simulink model "B1_quadcopter_model"  (R2021b)
settings: Solver=VariableStepAuto  StartTime=0.0  StopTime=10  RelTol=1e-3
values from neighbouring files (symbols this model uses):
  K_act = 50    [A10_simple_plant.m]    (also in A11_setup_script_pprz.m = 20; A1_setup_script.m = 20)
  K_act_inner = K_act*eye(4)    [A11_setup_script_pprz.m]    (also in A1_setup_script.m)
  K_u_d = 2.5    [A11_setup_script_pprz.m]    (also in A1_setup_script.m = 7)
  K_v_d = 2.5    [A11_setup_script_pprz.m]    (also in A1_setup_script.m = 7)
  K_w_d = 2.5    [A11_setup_script_pprz.m]    (also in A1_setup_script.m = 7)
  max_motor_rate = 30000    [A11_setup_script_pprz.m]    (also in A1_setup_script.m)
  max_omega_motor = 11000    [A11_setup_script_pprz.m]    (also in A1_setup_script.m)
  omega_c_motors = 50    [A11_setup_script_pprz.m]    (also in A1_setup_script.m)
  sampling_time = 1/frequency    (= 0.002)    [A11_setup_script_pprz.m]    (also in A12_sim_multi_run.m; A1_setup_script.m; A6_slow_actuator.m)
undefined symbols (not defined in the file or in its folder): K_ec_d_p, K_ec_d_q, K_ec_d_r, K_ec_dd_p, K_ec_dd_q, K_ec_dd_r, K_ec_p, K_ec_q, K_ec_r, K_p, K_p_d, K_p_dd, K_q, K_q_d, K_q_dd, K_r, K_r_d, K_r_dd
libraries: dspinverses x11, simulink_extras x6, sim3dlib x1, uavsim3dlib x1, vrlib x1, aerolibutil x1, sharedutil x1, aerolibbdyn x1, aerolibatmos2 x1
(part 1 of 3)
settings Model: Creator=pieca  LastModifiedBy=pieca

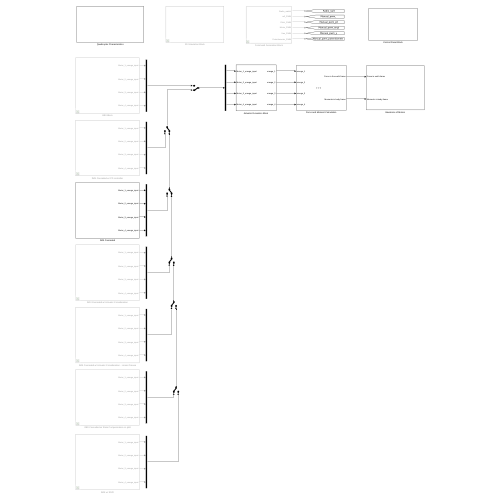
[thumbnail: Simulink's stored preview of the top-level diagram]
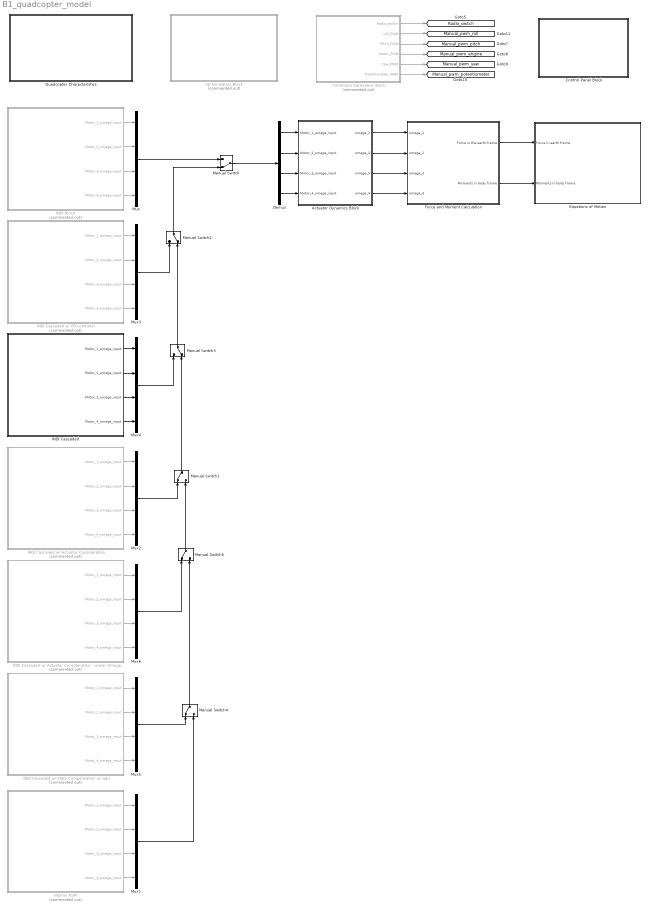
== system B1_quadcopter_model ==
  3D Simulation Block : Subsystem  Commented=on
  Actuator Dynamics Block : Subsystem
  Command Generation Block : Subsystem  Commented=on
  Control Panel Block : Subsystem
  Demux : Demux
  Equations of Motion : Subsystem
  Force and Moment Calculation : Subsystem
      mask Display: image('C:\Users\pieca\Desktop\AE5310-Thesis-Control\Quadcopter\media\bebop.jpg'); % Use "Edit Image" on toolstrip to change.
  INDI Block : Subsystem  Commented=on
  INDI Cascaded : Subsystem
  INDI Cascaded w/ Actuator Consideration : Subsystem  Commented=on
  INDI Cascaded w/ Actuator Consideration - Linear Omega : Subsystem  Commented=on
  INDI Cascaded w/ PD controller : Subsystem  Commented=on
  INDI Cascaded w/ State Compensation on qdd : Subsystem  Commented=on
  INDI w/ RSPI : Subsystem  Commented=on
  Manual Switch : ManualSwitch  CurrentSetting=0
  Manual Switch1 : ManualSwitch
  Manual Switch2 : ManualSwitch  CurrentSetting=0
  Manual Switch3 : ManualSwitch  CurrentSetting=0
  Manual Switch4 : ManualSwitch
  Manual Switch5 : ManualSwitch
  Mux{,1..6} (7 alike) : Mux
  Quadcopter Characteristics : Subsystem
  tag scope: Manual_pwm_engine=global, Manual_pwm_pitch=global, Manual_pwm_potentiometer=global, Manual_pwm_roll=global, Manual_pwm_yaw=global, Radio_switch=global
  wires:
  Command Generation Block/1(Radio_switch) -> [Radio_switch]
  Command Generation Block/2(roll_PWM) -> [Manual_pwm_roll]
  Command Generation Block/3(Pitch_PWM) -> [Manual_pwm_pitch]
  Command Generation Block/4(Motor_PWM) -> [Manual_pwm_engine]
  Command Generation Block/5(Yaw_PWM) -> [Manual_pwm_yaw]
  Command Generation Block/6(Potentiometer_PWM) -> [Manual_pwm_potentiometer]
  INDI Block/1(Motor_1_omega_input) -> Mux/1
  INDI Block/2(Motor_2_omega_input) -> Mux/2
  INDI Block/3(Motor_3_omega_input) -> Mux/3
  INDI Block/4(Motor_4_omega_input) -> Mux/4
  Demux/1 -> Actuator Dynamics Block/1(Motor_1_omega_input)
  Demux/2 -> Actuator Dynamics Block/2(Motor_2_omega_input)
  Demux/3 -> Actuator Dynamics Block/3(Motor_3_omega_input)
  Demux/4 -> Actuator Dynamics Block/4(Motor_4_omega_input)
  Force and Moment Calculation/1(Force in the earth frame) -> Equations of Motion/1(Force in earth frame)
  Force and Moment Calculation/2(Moments in body frame) -> Equations of Motion/2(Moments in body frame)
  Actuator Dynamics Block/1(omega_1) -> Force and Moment Calculation/1(omega_1)
  Actuator Dynamics Block/2(omega_2) -> Force and Moment Calculation/2(omega_2)
  Actuator Dynamics Block/3(omega_3) -> Force and Moment Calculation/3(omega_3)
  Actuator Dynamics Block/4(omega_4) -> Force and Moment Calculation/4(omega_4)
  INDI w/ RSPI/3(Motor_3_omega_input) -> Mux1/3
  INDI w/ RSPI/4(Motor_4_omega_input) -> Mux1/4
  INDI w/ RSPI/2(Motor_2_omega_input) -> Mux1/2
  INDI w/ RSPI/1(Motor_1_omega_input) -> Mux1/1
  Mux/1 -> Manual Switch/1
  Manual Switch/1 -> Demux/1
  INDI Cascaded w/ Actuator Consideration/4(Motor_4_omega_input) -> Mux2/4
  INDI Cascaded w/ Actuator Consideration/1(Motor_1_omega_input) -> Mux2/1
  INDI Cascaded w/ Actuator Consideration/2(Motor_2_omega_input) -> Mux2/2
  INDI Cascaded w/ Actuator Consideration/3(Motor_3_omega_input) -> Mux2/3
  Mux2/1 -> Manual Switch1/1
  INDI Cascaded w/ PD controller/2(Motor_2_omega_input) -> Mux3/2
  INDI Cascaded w/ PD controller/3(Motor_3_omega_input) -> Mux3/3
  INDI Cascaded w/ PD controller/1(Motor_1_omega_input) -> Mux3/1
  INDI Cascaded w/ PD controller/4(Motor_4_omega_input) -> Mux3/4
  Manual Switch2/1 -> Manual Switch/2
  Mux3/1 -> Manual Switch2/1
  INDI Cascaded/4(Motor_4_omega_input) -> Mux4/4
  INDI Cascaded/3(Motor_3_omega_input) -> Mux4/3
  INDI Cascaded/2(Motor_2_omega_input) -> Mux4/2
  INDI Cascaded/1(Motor_1_omega_input) -> Mux4/1
  Manual Switch1/1 -> Manual Switch3/2
  Manual Switch3/1 -> Manual Switch2/2
  Mux4/1 -> Manual Switch3/1
  INDI Cascaded w/ State Compensation on qdd/3(Motor_3_omega_input) -> Mux5/3
  INDI Cascaded w/ State Compensation on qdd/4(Motor_4_omega_input) -> Mux5/4
  INDI Cascaded w/ State Compensation on qdd/1(Motor_1_omega_input) -> Mux5/1
  INDI Cascaded w/ State Compensation on qdd/2(Motor_2_omega_input) -> Mux5/2
  Mux5/1 -> Manual Switch4/1
  Mux1/1 -> Manual Switch4/2
  INDI Cascaded w/ Actuator Consideration - Linear Omega/2(Motor_2_omega_input) -> Mux6/2
  INDI Cascaded w/ Actuator Consideration - Linear Omega/4(Motor_4_omega_input) -> Mux6/4
  INDI Cascaded w/ Actuator Consideration - Linear Omega/3(Motor_3_omega_input) -> Mux6/3
  INDI Cascaded w/ Actuator Consideration - Linear Omega/1(Motor_1_omega_input) -> Mux6/1
  Mux6/1 -> Manual Switch5/1
  Manual Switch4/1 -> Manual Switch5/2
  Manual Switch5/1 -> Manual Switch1/2

== system B1_quadcopter_model/3D Simulation Block ==
  Demux : Demux  Outputs=3
  Gain{,1..3} (4 alike) : Gain  Gain=-1
  Simulation 3D Scene Configuration : sim3dlib/Simulation 3D Scene Configuration  Priority=0  ProjectFormat_internal=Default Scenes  ProjectFormat=Default Scenes  SceneDesc=US city block  ProjectName=C:\Program Files\MATLAB\R2021b\toolbox\shared\sim3d_projects\automotive_project\UE4\WindowsNoEditor\VehicleSimulation.exe  ScenePath=/Game/Maps/USCityBlock  vehTagList={'Scene Origin';'SimulinkVehicle1'}  vehTag=SimulinkVehicle1  OpVisEn=off  Ts=0.08  EnableWindow=on  EnableWeather=off  SunAltitude=40.0  SunAzimuth=90  clouds=10  wind=1  fog=0  rain=0  sensorTag=MainCamera1  sensorId=1  sensorName=MainCamera1  mountLoc=Origin  offsetFlag=off  tmountOffset=[0, 0, 0]  rmountOffset=[0, 0, 0]  HorizontalResolution=1280  VerticalResolution=720  HorizontalFOV=60  mountPoint=[0 0 0]  mountOrientation=[0 0 0]  aMode=4  ID=1
      settings: SourceProductBaseCode=AE,DR,UV,VE
  Simulation 3D UAV Vehicle1 : uavsim3dlib/Simulation 3D UAV Vehicle  Priority=-1  Mesh=Quadrotor  MeshPath=mesh\Fixed_Wing_UAV.stl  Color=Red  ActorName=SimulinkVehicle1  InitialTranslation=[0 0 0]  InitialRotation=[0 0 0]  SampleTime=-1  ActorType=SimulinkVehicle  ID=1  aMode=4  ActorTag=SimulinkVehicle1
      settings: SourceProductBaseCode=UV
  Vector Concatenate : Concatenate  NumInputs=3
  Vector Concatenate1 : Concatenate  NumInputs=3
  wires:
  Gain1/1 -> Vector Concatenate1/2
  [x_earth] -> Vector Concatenate1/1
  [z_earth] -> Gain/1
  Gain3/1 -> Vector Concatenate/1
  Demux/1 -> Vector Concatenate/3
  Gain/1 -> Vector Concatenate1/3
  Demux/2 -> Gain2/1
  [y_earth] -> Gain1/1
  [PhiThetaPsi] -> Demux/1
  Vector Concatenate1/1 -> Simulation 3D UAV Vehicle1/1
  Demux/3 -> Gain3/1
  Vector Concatenate/1 -> Simulation 3D UAV Vehicle1/2
  Gain2/1 -> Vector Concatenate/2

== system B1_quadcopter_model/Actuator Dynamics Block ==
  Motor_1_omega_input : Inport
  Motor_2_omega_input : Inport  Port=2
  Motor_3_omega_input : Inport  Port=3
  Motor_4_omega_input : Inport  Port=4
  Clock : Clock
  Constant : Constant  Value=.1
  Constant1 : Constant  Value=1000
  Constant2 : Constant  Value=1000
  Display : Display
  Display1 : Display
  Saturation{1..4} (4 alike) : Saturate  UpperLimit=max_omega_motor  LowerLimit=10
  Sum : Sum  Inputs=|+-
  Switch{,1..3} (4 alike) : Switch  Criteria=u2 > Threshold
  Transfer Fcn{,1..3} (4 alike) : TransferFcn  Numerator=[omega_c_motors]  Denominator=[1 omega_c_motors]
  omega_1 : Outport
  omega_2 : Outport  Port=2
  omega_3 : Outport  Port=3
  omega_4 : Outport  Port=4
  wires:
  Sum/1 -> Switch3/2, Switch2/2, Switch1/2, Switch/2
  Constant1/1 -> Switch/3, Switch1/3
  Switch1/1 -> omega_2/1
  Transfer Fcn2/1 -> Switch2/1  "omega_3"
  Constant/1 -> Sum/2
  Motor_3_omega_input/1 -> Saturation2/1  "omega_3_in"
  Constant2/1 -> Switch2/3, Switch3/3
  Switch3/1 -> omega_4/1
  Transfer Fcn/1 -> Display1/1, Switch/1  "omega_1"
  Motor_4_omega_input/1 -> Saturation3/1  "omega_4_in"
  Saturation1/1 -> Transfer Fcn1/1
  Transfer Fcn3/1 -> Switch3/1  "omega_4"
  Switch/1 -> omega_1/1
  Saturation2/1 -> Transfer Fcn2/1
  Saturation3/1 -> Transfer Fcn3/1
  Saturation4/1 -> Transfer Fcn/1
  Transfer Fcn1/1 -> Switch1/1  "omega_2"
  Motor_2_omega_input/1 -> Saturation1/1  "omega_2_in"
  Motor_1_omega_input/1 -> Display/1, Saturation4/1  "omega_1_in"
  Clock/1 -> Sum/1
  Switch2/1 -> omega_3/1

== system B1_quadcopter_model/Command Generation Block ==
  note: Mapping Scheme (PWM)
      |
      | - roll: 1000 to 2000
      | - pitch: 1000 to 2000
      | - engine: 500 to 1500
      | - yaw: 1000 to 2000
      | - potent: 1000 to 2000
  note: Control Mapping for FlySky Controller
  Constant : Constant  Value=1500
  Constant1 : Constant  Value=1000
  Demux : Demux  Outputs=6
  Display{,1..7,9..10} (10 alike) : Display
  Gain{,2..3,5} (4 alike) : Gain  Gain=500
  Gain1 : Gain  Gain=-500
  Gain{4,6..9} (5 alike) : Gain  Gain=1/0.75
  Joystick Input : vrlib/Joystick Input  joyid=1  adjustports=on  forcefeed=off
  Selector : Selector  InputPortWidth=16  IndexOptions=Index vector (dialog)  Indices=1  OutputSizes=1
  Sum{,1..3,5} (5 alike) : Sum  Inputs=|++
  Terminator : Terminator
  Radio_switch : Outport
  roll_PWM : Outport  Port=2
  Pitch_PWM : Outport  Port=3
  Motor_PWM : Outport  Port=4
  Yaw_PWM : Outport  Port=5
  Potentiometer_PWM : Outport  Port=6
  wires:
  Gain2/1 -> Sum2/1
  Joystick Input/2 -> Selector/1
  Gain1/1 -> Sum1/1
  Sum/1 -> roll_PWM/1, Display4/1  "PWM roll"
  Constant1/1 -> Sum2/2
  Selector/1 -> Radio_switch/1  "Switch value"
  Gain5/1 -> Sum5/1
  Joystick Input/1 -> Demux/1
  Sum3/1 -> Yaw_PWM/1, Display7/1  "PWM Yaw"
  Sum5/1 -> Display10/1  "PWM potentiometer"
  Demux/1 -> Display/1, Gain4/1  "roll"
  Demux/2 -> Gain6/1, Display1/1  "pitch"
  Demux/5 -> Gain8/1, Display9/1  "potentiometer"
  Constant/1 -> Sum5/2, Sum/2, Sum1/2, Sum3/2
  Sum2/1 -> Motor_PWM/1, Display6/1  "PWM engine"
  Sum1/1 -> Pitch_PWM/1, Display5/1  "PWM pitch"
  Gain/1 -> Sum/1
  Demux/4 -> Gain9/1, Display3/1  "Yaw"
  Gain3/1 -> Sum3/1
  Demux/3 -> Gain7/1, Display2/1  "engine"
  Demux/6 -> Terminator/1
  Gain6/1 -> Gain1/1
  Gain9/1 -> Gain3/1
  Gain7/1 -> Gain2/1
  Gain4/1 -> Gain/1
  Gain8/1 -> Gain5/1

== system B1_quadcopter_model/Control Panel Block ==
  note: Desired state in the Earth Frame
  " " : SliderBlock  ScaleMin=500  ScaleMax=1500
  Demux : Demux  Outputs=3
  Disturbance Block : Subsystem
  Gain : Gain  Gain=0.006
  Gain1 : Gain  Gain=0.006
  Gain2 : Gain  Gain=-0.006
  Gain3 : Gain  Gain=0.004
  Gain4 : Gain  Gain=-1
  Horizontal : Display
  Horizontal Slider1 : SliderBlock  ScaleMin=1000  ScaleMax=2000
  Horizontal Slider2 : SliderBlock  ScaleMin=1000  ScaleMax=2000
  Horizontal Slider3 : SliderBlock  ScaleMin=1000  ScaleMax=2000
  Horizontal Speed : Constant  Value=1000.392587939699
  Integrator : Integrator
  Lateral : Display
  Lateral Speed : Constant  Value=1500
  Manual Switch{,1..3} (4 alike) : ManualSwitch  CurrentSetting=0
  MatrixMultiply : Product  Multiplication=Matrix(*)
  PWM Attitude : Constant  Value=1500
  PWM Engine : Constant  Value=1000
  Scope : Scope  NumInputPorts=4
  Sum{,1..3} (4 alike) : Sum  Inputs=|+-
  Sum4 : Sum  Inputs=|++
  Sum5 : Sum  Inputs=|++
  Sum6 : Sum  Inputs=|++
  Vector Concatenate : Concatenate  NumInputs=3
  Vertical : Display
  Vertical Speed : Constant  Value=1500
  Yaw Angle Change : Constant  Value=1500
  Yaw Speed : Display
  tag scope: u_des=global, v_des=global, w_des=global, yaw_des=global
  wires:
  [Manual_pwm_roll] -> Manual Switch1/1
  Manual Switch3/1 -> Scope/4, Sum3/1
  [Manual_pwm_yaw] -> Manual Switch3/1
  Sum/1 -> Gain/1
  Gain/1 -> Horizontal/1, Vector Concatenate/1
  PWM Attitude/1 -> Sum3/2, Sum2/2, Sum1/2
  Horizontal Speed/1 -> Manual Switch/2
  Sum1/1 -> Gain1/1
  Yaw Angle Change/1 -> Manual Switch3/2
  Lateral Speed/1 -> Manual Switch1/2
  Vertical Speed/1 -> Manual Switch2/2
  Manual Switch/1 -> Scope/1, Sum/1
  Manual Switch1/1 -> Scope/2, Sum1/1
  Manual Switch2/1 -> Scope/3, Sum2/1
  Sum2/1 -> Gain2/1
  Sum3/1 -> Gain3/1
  Gain2/1 -> Vector Concatenate/3, Vertical/1
  [Manual_pwm_engine] -> Manual Switch/1
  [Manual_pwm_pitch] -> Manual Switch2/1
  PWM Engine/1 -> Sum/2
  Gain1/1 -> Lateral/1, Vector Concatenate/2
  [R_bg] -> MatrixMultiply/1
  Vector Concatenate/1 -> MatrixMultiply/2
  MatrixMultiply/1 -> Demux/1
  Gain3/1 -> Integrator/1, Yaw Speed/1
  Demux/1 -> Sum4/1
  Sum4/1 -> [u_des]
  Demux/2 -> Sum5/1
  Sum5/1 -> [v_des]
  Sum6/1 -> [w_des]
  Demux/3 -> Sum6/1
  Integrator/1 -> [yaw_des]
  Disturbance Block/1(Total Disturbance) -> Sum4/2, Gain4/1
  Gain4/1 -> Sum6/2

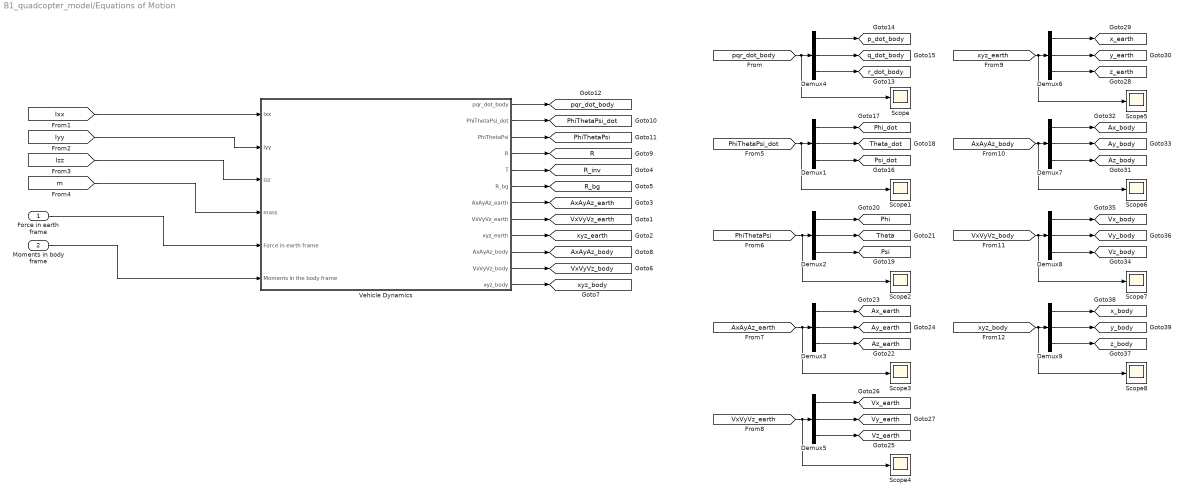
== system B1_quadcopter_model/Equations of Motion ==
  Force in earth frame : Inport
  Moments in body frame : Inport  Port=2
  Demux{1..9} (9 alike) : Demux  Outputs=3
  Scope{,1..8} (9 alike) : Scope
  Vehicle Dynamics : Subsystem
  tag scope: AxAyAz_body=global, AxAyAz_earth=global, Ax_body=global, Ax_earth=global, Ay_body=global, Ay_earth=global, Az_body=global, Az_earth=global, Phi=global, PhiThetaPsi=global, PhiThetaPsi_dot=global, Phi_dot=global, Psi=global, Psi_dot=global, R=global, R_bg=global, R_inv=global, Theta=global, Theta_dot=global, VxVyVz_body=global, VxVyVz_earth=global, Vx_body=global, Vx_earth=global, Vy_body=global, Vy_earth=global, Vz_body=global, Vz_earth=global, p_dot_body=global, pqr_dot_body=global, q_dot_body=global, r_dot_body=global, x_body=global, x_earth=global, xyz_body=global, xyz_earth=global, y_body=global, y_earth=global, z_body=global, z_earth=global
  wires:
  Force in earth frame/1 -> Vehicle Dynamics/5(Force in earth frame)
  Moments in body frame/1 -> Vehicle Dynamics/6(Moments in the body frame)
  [m] -> Vehicle Dynamics/4(mass)
  [Izz] -> Vehicle Dynamics/3(Izz)
  [Iyy] -> Vehicle Dynamics/2(Iyy)
  [Ixx] -> Vehicle Dynamics/1(Ixx)
  Vehicle Dynamics/5(T) -> [R_inv]
  Vehicle Dynamics/4(R) -> [R]
  Vehicle Dynamics/6(R_bg) -> [R_bg]
  Vehicle Dynamics/1(pqr_dot_body) -> [pqr_dot_body]
  Vehicle Dynamics/2(PhiThetaPsi_dot) -> [PhiThetaPsi_dot]
  Vehicle Dynamics/3(PhiThetaPsi) -> [PhiThetaPsi]
  Vehicle Dynamics/7(AxAyAz_earth) -> [AxAyAz_earth]
  Vehicle Dynamics/8(VxVyVz_earth) -> [VxVyVz_earth]
  Vehicle Dynamics/9(xyz_earth) -> [xyz_earth]
  Vehicle Dynamics/10(AxAyAz_body) -> [AxAyAz_body]
  Vehicle Dynamics/11(VxVyVz_body) -> [VxVyVz_body]
  Vehicle Dynamics/12(xyz_body) -> [xyz_body]
  Demux4/1 -> [p_dot_body]
  Demux4/3 -> [r_dot_body]
  [pqr_dot_body] -> Scope/1, Demux4/1
  Demux4/2 -> [q_dot_body]
  Demux1/2 -> [Theta_dot]
  Demux1/3 -> [Psi_dot]
  Demux1/1 -> [Phi_dot]
  [PhiThetaPsi] -> Scope2/1, Demux2/1
  Demux2/2 -> [Theta]
  Demux2/3 -> [Psi]
  Demux2/1 -> [Phi]
  Demux3/2 -> [Ay_earth]
  Demux3/1 -> [Ax_earth]
  Demux3/3 -> [Az_earth]
  [AxAyAz_earth] -> Scope3/1, Demux3/1
  Demux5/2 -> [Vy_earth]
  Demux5/1 -> [Vx_earth]
  Demux5/3 -> [Vz_earth]
  [VxVyVz_earth] -> Scope4/1, Demux5/1
  Demux6/2 -> [y_earth]
  Demux6/1 -> [x_earth]
  Demux6/3 -> [z_earth]
  [xyz_earth] -> Scope5/1, Demux6/1
  Demux7/2 -> [Ay_body]
  Demux7/1 -> [Ax_body]
  Demux7/3 -> [Az_body]
  [AxAyAz_body] -> Scope6/1, Demux7/1
  Demux8/2 -> [Vy_body]
  Demux8/1 -> [Vx_body]
  Demux8/3 -> [Vz_body]
  [VxVyVz_body] -> Scope7/1, Demux8/1
  Demux9/2 -> [y_body]
  Demux9/1 -> [x_body]
  Demux9/3 -> [z_body]
  [xyz_body] -> Scope8/1, Demux9/1
  [PhiThetaPsi_dot] -> Scope1/1, Demux1/1

== system B1_quadcopter_model/Force and Moment Calculation ==
  omega_1 : Inport
  omega_2 : Inport  Port=2
  omega_3 : Inport  Port=3
  omega_4 : Inport  Port=4
  Add : Sum
  Add1 : Sum
  Demux : Demux  Outputs=3
  Demux1 : Demux  Outputs=3
  Forces : Scope  NumInputPorts=3
  Forces and Moments due to Aerodynamic Forces : Subsystem
  Forces due to thrust : MATLAB Function  TreatAsAtomicUnit=on
  Moments : Scope  NumInputPorts=3
  Moments due to thrust : MATLAB Function  TreatAsAtomicUnit=on
  Scope : Scope
  Force in the earth frame : Outport
  Moments in body frame : Outport  Port=2
  tag scope: Fx_earth=global, Fy_earth=global, Fz_earth=global, Mx=global, My=global, Mz=global, T=global, omega_1=global, omega_2=global, omega_3=global, omega_4=global
  wires:
  omega_1/1 -> [omega_1]
  omega_4/1 -> [omega_4]
  omega_3/1 -> [omega_3]
  omega_2/1 -> [omega_2]
  [omega_4] -> Forces due to thrust/4(omega_4)
  [omega_3] -> Forces due to thrust/3(omega_3)
  [omega_2] -> Forces due to thrust/2(omega_2)
  [omega_1] -> Forces due to thrust/1(omega_1)
  [R_bg] -> Forces due to thrust/5(R_bg)
  [K_t] -> Forces due to thrust/6(K_t)
  Forces due to thrust/1(F_t_e) -> Forces/2, Add/2  "thrust_force"
  Add/1 -> Forces/3, Force in the earth frame/1, Demux/1  "total_force"
  [R_bg] -> Forces and Moments due to Aerodynamic Forces/2(R_bg)
  [z_earth] -> Forces and Moments due to Aerodynamic Forces/1(z_earth)
  Forces and Moments due to Aerodynamic Forces/1(F_aero) -> Forces/1  "aero_force"
  Moments due to thrust/1(M_t) -> Moments/2, Add1/2, Scope/1  "thrust_moment"
  [omega_1] -> Moments due to thrust/1(omega_1)
  [omega_2] -> Moments due to thrust/2(omega_2)
  [omega_3] -> Moments due to thrust/3(omega_3)
  [omega_4] -> Moments due to thrust/4(omega_4)
  [K_t] -> Moments due to thrust/5(K_t)
  [K_m] -> Moments due to thrust/6(K_m)
  Add1/1 -> Moments/3, Moments in body frame/1, Demux1/1  "full_moment"
  Demux/1 -> [Fx_earth]
  Demux/3 -> [Fz_earth]
  Demux/2 -> [Fy_earth]
  Demux1/2 -> [My]
  Demux1/1 -> [Mx]
  Demux1/3 -> [Mz]
  Forces due to thrust/2(F_t_b) -> [T]
  [b] -> Moments due to thrust/7(b)
  [l] -> Moments due to thrust/8(l)
  Forces and Moments due to Aerodynamic Forces/2(M_aero) -> Moments/1  "aero_moment"

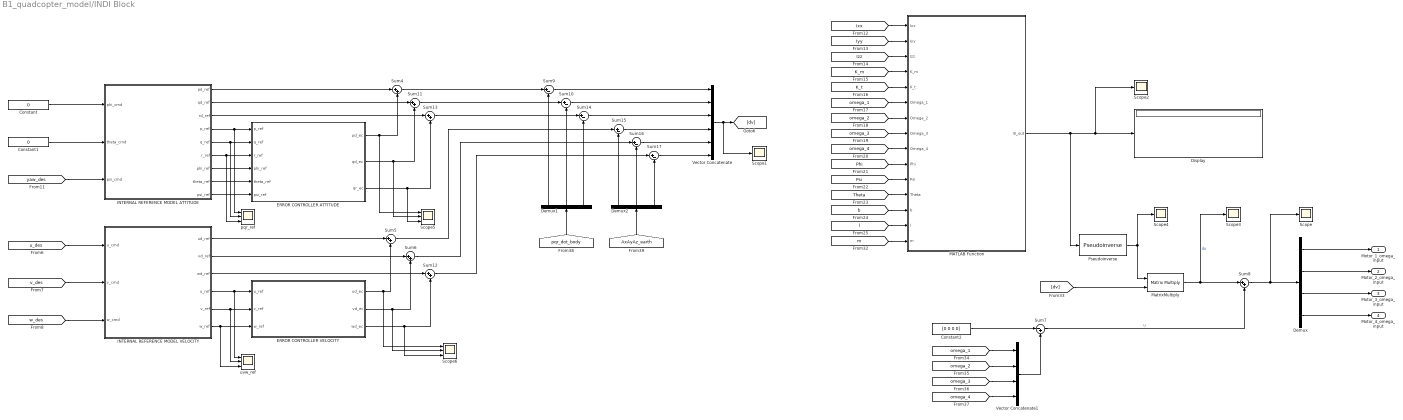
== system B1_quadcopter_model/INDI Block ==
  Constant : Constant  Value=0
  Constant1 : Constant  Value=0
  Constant2 : Constant  Value=[0 0 0 0]
  Demux : Demux
  Demux1 : Demux  Outputs=3
  Demux2 : Demux  Outputs=3
  Display : Display
  ERROR CONTROLLER ATTITUDE : Subsystem
  ERROR CONTROLLER VELOCITY : Subsystem
  INTERNAL REFERENCE MODEL ATTITUDE : Subsystem
  INTERNAL REFERENCE MODEL VELOCITY : Subsystem
  MATLAB Function : MATLAB Function  TreatAsAtomicUnit=on
  MatrixMultiply : Product  Multiplication=Matrix(*)
  Pseudoinverse : dspinverses/Pseudoinverse  wanterr=off  SimulateUsing=Interpreted execution
      settings: SourceProductBaseCode=DS
  Scope{,1..4} (5 alike) : Scope
  Scope5 : Scope  NumInputPorts=3
  Scope6 : Scope  NumInputPorts=3
  Sum{9..10,14..17} (6 alike) : Sum  Inputs=|+-
  Sum{4..6,8,11..13} (7 alike) : Sum  Inputs=|++
  Sum7 : Sum  Inputs=|-+
  Vector Concatenate : Concatenate  NumInputs=6
  Vector Concatenate1 : Concatenate  NumInputs=4
  pqr_ref : Scope  NumInputPorts=3
  uvw_ref : Scope  NumInputPorts=3
  Motor_1_omega_input : Outport
  Motor_2_omega_input : Outport  Port=2
  Motor_3_omega_input : Outport  Port=3
  Motor_4_omega_input : Outport  Port=4
  wires:
  ERROR CONTROLLER ATTITUDE/2(qd_ec) -> Scope5/2, Sum11/2
  INTERNAL REFERENCE MODEL ATTITUDE/2(qd_ref) -> Sum11/1
  INTERNAL REFERENCE MODEL ATTITUDE/1(pd_ref) -> Sum4/1
  INTERNAL REFERENCE MODEL ATTITUDE/5(q_ref) -> ERROR CONTROLLER ATTITUDE/2(q_ref), pqr_ref/2
  INTERNAL REFERENCE MODEL ATTITUDE/9(psi_ref) -> ERROR CONTROLLER ATTITUDE/6(psi_ref)
  INTERNAL REFERENCE MODEL ATTITUDE/6(r_ref) -> ERROR CONTROLLER ATTITUDE/3(r_ref), pqr_ref/3
  INTERNAL REFERENCE MODEL ATTITUDE/4(p_ref) -> pqr_ref/1, ERROR CONTROLLER ATTITUDE/1(p_ref)
  INTERNAL REFERENCE MODEL ATTITUDE/3(rd_ref) -> Sum13/1
  ERROR CONTROLLER ATTITUDE/3(qr_ec) -> Scope5/3, Sum13/2
  INTERNAL REFERENCE MODEL ATTITUDE/7(phi_ref) -> ERROR CONTROLLER ATTITUDE/4(phi_ref)
  ERROR CONTROLLER ATTITUDE/1(pd_ec) -> Scope5/1, Sum4/2
  INTERNAL REFERENCE MODEL ATTITUDE/8(theta_ref) -> ERROR CONTROLLER ATTITUDE/5(theta_ref)
  ERROR CONTROLLER VELOCITY/1(ud_ec) -> Scope6/1, Sum5/2
  ERROR CONTROLLER VELOCITY/3(wd_ec) -> Scope6/3, Sum12/2
  INTERNAL REFERENCE MODEL VELOCITY/3(wd_ref) -> Sum12/1
  INTERNAL REFERENCE MODEL VELOCITY/2(vd_ref) -> Sum6/1
  INTERNAL REFERENCE MODEL VELOCITY/5(v_ref) -> ERROR CONTROLLER VELOCITY/2(v_ref), uvw_ref/2
  Sum12/1 -> Sum17/1
  INTERNAL REFERENCE MODEL VELOCITY/6(w_ref) -> ERROR CONTROLLER VELOCITY/3(w_ref), uvw_ref/3
  Sum5/1 -> Sum15/1
  INTERNAL REFERENCE MODEL VELOCITY/1(ud_ref) -> Sum5/1
  ERROR CONTROLLER VELOCITY/2(vd_ec) -> Scope6/2, Sum6/2
  INTERNAL REFERENCE MODEL VELOCITY/4(u_ref) -> uvw_ref/1, ERROR CONTROLLER VELOCITY/1(u_ref)
  Sum6/1 -> Sum16/1
  [u_des] -> INTERNAL REFERENCE MODEL VELOCITY/1(u_cmd)
  [v_des] -> INTERNAL REFERENCE MODEL VELOCITY/2(v_cmd)
  [w_des] -> INTERNAL REFERENCE MODEL VELOCITY/3(w_cmd)
  Constant/1 -> INTERNAL REFERENCE MODEL ATTITUDE/1(phi_cmd)
  Constant1/1 -> INTERNAL REFERENCE MODEL ATTITUDE/2(theta_cmd)
  [yaw_des] -> INTERNAL REFERENCE MODEL ATTITUDE/3(psi_cmd)
  Sum4/1 -> Sum9/1
  Sum11/1 -> Sum10/1
  Sum13/1 -> Sum14/1
  Vector Concatenate/1 -> Scope1/1, [dv]
  [Ixx] -> MATLAB Function/1(Ixx)
  [Iyy] -> MATLAB Function/2(Iyy)
  [Izz] -> MATLAB Function/3(Izz)
  [K_m] -> MATLAB Function/4(K_m)
  [K_t] -> MATLAB Function/5(K_t)
  [omega_1] -> MATLAB Function/6(Omega_1)
  [omega_2] -> MATLAB Function/7(Omega_2)
  [omega_3] -> MATLAB Function/8(Omega_3)
  [omega_4] -> MATLAB Function/9(Omega_4)
  [Phi] -> MATLAB Function/10(Phi)
  [Psi] -> MATLAB Function/11(Psi)
  [Theta] -> MATLAB Function/12(Theta)
  [b] -> MATLAB Function/13(b)
  [l] -> MATLAB Function/14(l)
  [m] -> MATLAB Function/15(m)
  MATLAB Function/1(B_out) -> Pseudoinverse/1, Scope2/1, Display/1
  Pseudoinverse/1 -> MatrixMultiply/1, Scope4/1
  MatrixMultiply/1 -> Scope3/1, Sum8/1  "du"
  [omega_1] -> Vector Concatenate1/1
  [omega_2] -> Vector Concatenate1/2
  [omega_3] -> Vector Concatenate1/3
  [omega_4] -> Vector Concatenate1/4
  Vector Concatenate1/1 -> Sum7/2
  Constant2/1 -> Sum7/1
  Sum7/1 -> Sum8/2  "u"
  Sum8/1 -> Scope/1, Demux/1
  Demux/1 -> Motor_1_omega_input/1
  Demux/2 -> Motor_2_omega_input/1
  Demux/3 -> Motor_3_omega_input/1
  Demux/4 -> Motor_4_omega_input/1
  Sum9/1 -> Vector Concatenate/1
  Sum10/1 -> Vector Concatenate/2
  Sum14/1 -> Vector Concatenate/3
  Sum15/1 -> Vector Concatenate/4
  Sum16/1 -> Vector Concatenate/5
  Sum17/1 -> Vector Concatenate/6
  [pqr_dot_body] -> Demux1/1
  [AxAyAz_earth] -> Demux2/1
  Demux2/3 -> Sum17/2
  Demux2/2 -> Sum16/2
  Demux2/1 -> Sum15/2
  Demux1/3 -> Sum14/2
  Demux1/2 -> Sum10/2
  Demux1/1 -> Sum9/2
  [dv] -> MatrixMultiply/2

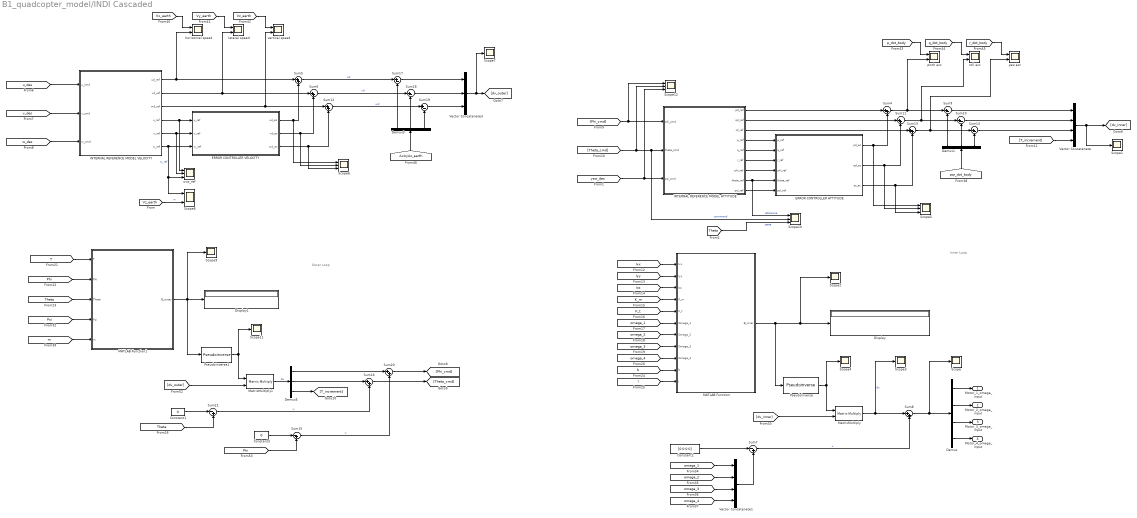
== system B1_quadcopter_model/INDI Cascaded ==
  note: Outer Loop
  note: Inner Loop
  Constant1 : Constant  Value=0
  Constant2 : Constant  Value=[0 0 0 0]
  Constant3 : Constant  Value=0
  Demux : Demux
  Demux1 : Demux  Outputs=3
  Demux3 : Demux  Outputs=3
  Demux5 : Demux  Outputs=3
  Display : Display
  Display1 : Display
  ERROR CONTROLLER ATTITUDE : Subsystem
  ERROR CONTROLLER VELOCITY : Subsystem
  INTERNAL REFERENCE MODEL ATTITUDE : Subsystem
  INTERNAL REFERENCE MODEL VELOCITY : Subsystem
  MATLAB Function : MATLAB Function  TreatAsAtomicUnit=on
  MATLAB Function1 : MATLAB Function  TreatAsAtomicUnit=on
  MatrixMultiply : Product  Multiplication=Matrix(*)
  MatrixMultiply1 : Product  Multiplication=Matrix(*)
  Pseudoinverse : dspinverses/Pseudoinverse  wanterr=off  SimulateUsing=Interpreted execution
      settings: SourceProductBaseCode=DS
  Pseudoinverse1 : dspinverses/Pseudoinverse  wanterr=off  SimulateUsing=Interpreted execution
      settings: SourceProductBaseCode=DS
  Scope{,1..4,7,9,11} (8 alike) : Scope
  Scope{5..6,10,12} (4 alike) : Scope  NumInputPorts=3
  Scope8 : Scope  NumInputPorts=2
  Sum{9..10,14,17..19} (6 alike) : Sum  Inputs=|+-
  Sum{4..6,8,11..13,16,20} (9 alike) : Sum  Inputs=|++
  Sum15 : Sum  Inputs=|-+
  Sum21 : Sum  Inputs=|-+
  Sum7 : Sum  Inputs=|-+
  Vector Concatenate : Concatenate  NumInputs=4
  Vector Concatenate1 : Concatenate  NumInputs=4
  Vector Concatenate3 : Concatenate  NumInputs=3
  horizontal speed : Scope  NumInputPorts=2
  lateral speed : Scope  NumInputPorts=2
  pitch acc : Scope  NumInputPorts=2
  roll acc : Scope  NumInputPorts=2
  uvw_ref : Scope  NumInputPorts=3
  vertical speed : Scope  NumInputPorts=2
  yaw acc : Scope  NumInputPorts=2
  Motor_1_omega_input : Outport
  Motor_2_omega_input : Outport  Port=2
  Motor_3_omega_input : Outport  Port=3
  Motor_4_omega_input : Outport  Port=4
  wires:
  ERROR CONTROLLER ATTITUDE/2(qd_ec) -> Sum11/2, Scope5/2
  INTERNAL REFERENCE MODEL ATTITUDE/2(qd_ref) -> Sum11/1
  INTERNAL REFERENCE MODEL ATTITUDE/1(pd_ref) -> Sum4/1
  INTERNAL REFERENCE MODEL ATTITUDE/5(q_ref) -> ERROR CONTROLLER ATTITUDE/2(q_ref)
  INTERNAL REFERENCE MODEL ATTITUDE/9(psi_ref) -> ERROR CONTROLLER ATTITUDE/6(psi_ref)
  INTERNAL REFERENCE MODEL ATTITUDE/6(r_ref) -> ERROR CONTROLLER ATTITUDE/3(r_ref)
  INTERNAL REFERENCE MODEL ATTITUDE/4(p_ref) -> ERROR CONTROLLER ATTITUDE/1(p_ref)
  INTERNAL REFERENCE MODEL ATTITUDE/3(rd_ref) -> Sum13/1
  ERROR CONTROLLER ATTITUDE/3(qr_ec) -> Sum13/2, Scope5/3
  INTERNAL REFERENCE MODEL ATTITUDE/7(phi_ref) -> ERROR CONTROLLER ATTITUDE/4(phi_ref)
  ERROR CONTROLLER ATTITUDE/1(pd_ec) -> Sum4/2, Scope5/1
  INTERNAL REFERENCE MODEL ATTITUDE/8(theta_ref) -> Scope10/1, ERROR CONTROLLER ATTITUDE/5(theta_ref)  "reference"
  ERROR CONTROLLER VELOCITY/1(ud_ec) -> Sum5/2, Scope6/1
  ERROR CONTROLLER VELOCITY/3(wd_ec) -> Sum12/2, Scope6/3
  INTERNAL REFERENCE MODEL VELOCITY/3(wd_ref) -> vertical speed/2, Sum12/1
  INTERNAL REFERENCE MODEL VELOCITY/2(vd_ref) -> lateral speed/2, Sum6/1
  INTERNAL REFERENCE MODEL VELOCITY/5(v_ref) -> ERROR CONTROLLER VELOCITY/2(v_ref), uvw_ref/2
  INTERNAL REFERENCE MODEL VELOCITY/6(w_ref) -> ERROR CONTROLLER VELOCITY/3(w_ref), Scope8/1, uvw_ref/3  "w_ref"
  INTERNAL REFERENCE MODEL VELOCITY/1(ud_ref) -> horizontal speed/2, Sum5/1
  ERROR CONTROLLER VELOCITY/2(vd_ec) -> Sum6/2, Scope6/2
  INTERNAL REFERENCE MODEL VELOCITY/4(u_ref) -> ERROR CONTROLLER VELOCITY/1(u_ref), uvw_ref/1
  [u_des] -> INTERNAL REFERENCE MODEL VELOCITY/1(u_cmd)
  [v_des] -> INTERNAL REFERENCE MODEL VELOCITY/2(v_cmd)
  [w_des] -> INTERNAL REFERENCE MODEL VELOCITY/3(w_cmd)
  [Phi_cmd] -> Scope12/1, INTERNAL REFERENCE MODEL ATTITUDE/1(phi_cmd)
  [Theta_cmd] -> Scope12/2, Scope10/2, INTERNAL REFERENCE MODEL ATTITUDE/2(theta_cmd)  "command"
  [yaw_des] -> Scope12/3, INTERNAL REFERENCE MODEL ATTITUDE/3(psi_cmd)
  Vector Concatenate/1 -> Scope1/1, [dv_inner]
  MATLAB Function/1(B_inner) -> Pseudoinverse/1, Scope2/1, Display/1
  Pseudoinverse/1 -> MatrixMultiply/1, Scope4/1
  MatrixMultiply/1 -> Scope3/1, Sum8/1  "du"
  [omega_1] -> Vector Concatenate1/1
  [omega_2] -> Vector Concatenate1/2
  [omega_3] -> Vector Concatenate1/3
  [omega_4] -> Vector Concatenate1/4
  Vector Concatenate1/1 -> Sum7/2
  Constant2/1 -> Sum7/1
  Sum7/1 -> Sum8/2  "u"
  Sum8/1 -> Scope/1, Demux/1
  Demux/1 -> Motor_1_omega_input/1
  Demux/2 -> Motor_2_omega_input/1
  Demux/3 -> Motor_3_omega_input/1
  Demux/4 -> Motor_4_omega_input/1
  Sum9/1 -> Vector Concatenate/1
  Sum10/1 -> Vector Concatenate/2
  Sum14/1 -> Vector Concatenate/3
  [pqr_dot_body] -> Demux1/1
  Demux1/3 -> Sum14/2
  Demux1/2 -> Sum10/2
  Demux1/1 -> Sum9/2
  [dv_inner] -> MatrixMultiply/2
  [T_increment] -> Vector Concatenate/4
  Sum4/1 -> pitch acc/2, Sum9/1
  Sum11/1 -> roll acc/2, Sum10/1
  Sum13/1 -> yaw acc/2, Sum14/1
  Sum12/1 -> Sum19/1  "wd"
  Sum6/1 -> Sum18/1  "vd"
  Sum5/1 -> Sum17/1  "ud"
  Vector Concatenate3/1 -> Scope7/1, [dv_outer]
  [Vz_earth] -> vertical speed/1
  [Vy_earth] -> lateral speed/1
  [Vx_earth] -> horizontal speed/1
  [r_dot_body] -> yaw acc/1
  [p_dot_body] -> pitch acc/1
  [q_dot_body] -> roll acc/1
  Sum19/1 -> Vector Concatenate3/3
  Sum18/1 -> Vector Concatenate3/2
  Sum17/1 -> Vector Concatenate3/1
  [AxAyAz_earth] -> Demux3/1
  Demux3/3 -> Sum19/2
  Demux3/2 -> Sum18/2
  Demux3/1 -> Sum17/2
  [K_m] -> MATLAB Function/4(K_m)
  [Izz] -> MATLAB Function/3(Izz)
  [Iyy] -> MATLAB Function/2(Iyy)
  [Ixx] -> MATLAB Function/1(Ixx)
  [omega_3] -> MATLAB Function/8(Omega_3)
  [omega_1] -> MATLAB Function/6(Omega_1)
  [omega_4] -> MATLAB Function/9(Omega_4)
  [K_t] -> MATLAB Function/5(K_t)
  [b] -> MATLAB Function/10(b)
  [l] -> MATLAB Function/11(l)
  [omega_2] -> MATLAB Function/7(Omega_2)
  Pseudoinverse1/1 -> Scope11/1, MatrixMultiply1/1
  Sum20/1 -> [Phi_cmd]
  Demux5/1 -> Sum20/1
  [Phi] -> MATLAB Function1/2(Phi)
  Demux5/2 -> Sum16/1
  MatrixMultiply1/1 -> Demux5/1  "du"
  Sum21/1 -> Sum16/2  "u"
  [Theta] -> Sum21/2
  [m] -> MATLAB Function1/5(m)
  [T] -> MATLAB Function1/1(T)
  [dv_outer] -> MatrixMultiply1/2
  Constant1/1 -> Sum21/1
  [Phi] -> Sum15/2
  Sum16/1 -> [Theta_cmd]
  [Psi] -> MATLAB Function1/4(Psi)
  [Theta] -> MATLAB Function1/3(Theta)
  Demux5/3 -> [T_increment]
  Sum15/1 -> Sum20/2  "u"
  MATLAB Function1/1(B_outer) -> Pseudoinverse1/1, Scope9/1, Display1/1
  Constant3/1 -> Sum15/1
  [Vz_earth] -> Scope8/2  "w"
  [Theta] -> Scope10/3  "state"

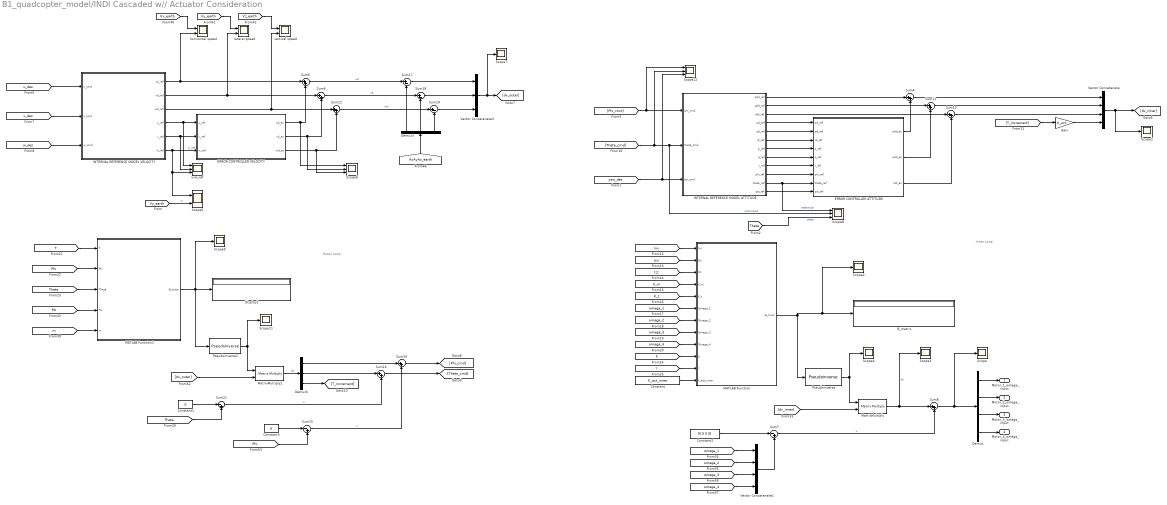
== system B1_quadcopter_model/INDI Cascaded w// Actuator Consideration ==
  note: Outer Loop
  note: Inner Loop
  B_matrix : Display
  Constant : Constant  Value=K_act_inner
  Constant1 : Constant  Value=0
  Constant2 : Constant  Value=[0 0 0 0]
  Constant3 : Constant  Value=0
  Demux : Demux
  Demux3 : Demux  Outputs=3
  Demux5 : Demux  Outputs=3
  Display1 : Display
  ERROR CONTROLLER ATTITUDE : Subsystem
  ERROR CONTROLLER VELOCITY : Subsystem
  Gain : Gain  Gain=K_act
  INTERNAL REFERENCE MODEL ATTITUDE : Subsystem
  INTERNAL REFERENCE MODEL VELOCITY : Subsystem
  MATLAB Function : MATLAB Function  TreatAsAtomicUnit=on
  MATLAB Function1 : MATLAB Function  TreatAsAtomicUnit=on
  MatrixMultiply : Product  Multiplication=Matrix(*)
  MatrixMultiply1 : Product  Multiplication=Matrix(*)
  Pseudoinverse : dspinverses/Pseudoinverse  wanterr=off  SimulateUsing=Interpreted execution
      settings: SourceProductBaseCode=DS
  Pseudoinverse1 : dspinverses/Pseudoinverse  wanterr=off  SimulateUsing=Interpreted execution
      settings: SourceProductBaseCode=DS
  Scope{,1..4,7,9,11} (8 alike) : Scope
  Scope12 : Scope  NumInputPorts=3
  Scope5 : Scope  NumInputPorts=2
  Scope6 : Scope  NumInputPorts=3
  Scope8 : Scope  NumInputPorts=3
  Sum{4..6,8,11..13,16,20} (9 alike) : Sum  Inputs=|++
  Sum15 : Sum  Inputs=|-+
  Sum17 : Sum  Inputs=|+-
  Sum18 : Sum  Inputs=|+-
  Sum19 : Sum  Inputs=|+-
  Sum21 : Sum  Inputs=|-+
  Sum7 : Sum  Inputs=|-+
  Vector Concatenate : Concatenate  NumInputs=4
  Vector Concatenate1 : Concatenate  NumInputs=4
  Vector Concatenate3 : Concatenate  NumInputs=3
  horizontal speed : Scope  NumInputPorts=2
  lateral speed : Scope  NumInputPorts=2
  uvw_ref : Scope  NumInputPorts=3
  vertical speed : Scope  NumInputPorts=2
  Motor_1_omega_input : Outport
  Motor_2_omega_input : Outport  Port=2
  Motor_3_omega_input : Outport  Port=3
  Motor_4_omega_input : Outport  Port=4
  wires:
  ERROR CONTROLLER VELOCITY/1(ud_ec) -> Sum5/2, Scope6/1
  ERROR CONTROLLER VELOCITY/3(wd_ec) -> Sum12/2, Scope6/3
  INTERNAL REFERENCE MODEL VELOCITY/3(wd_ref) -> vertical speed/2, Sum12/1
  INTERNAL REFERENCE MODEL VELOCITY/2(vd_ref) -> lateral speed/2, Sum6/1
  INTERNAL REFERENCE MODEL VELOCITY/5(v_ref) -> ERROR CONTROLLER VELOCITY/2(v_ref), uvw_ref/2
  INTERNAL REFERENCE MODEL VELOCITY/6(w_ref) -> ERROR CONTROLLER VELOCITY/3(w_ref), Scope5/1, uvw_ref/3  "w_ref"
  INTERNAL REFERENCE MODEL VELOCITY/1(ud_ref) -> horizontal speed/2, Sum5/1
  ERROR CONTROLLER VELOCITY/2(vd_ec) -> Sum6/2, Scope6/2
  INTERNAL REFERENCE MODEL VELOCITY/4(u_ref) -> ERROR CONTROLLER VELOCITY/1(u_ref), uvw_ref/1
  [u_des] -> INTERNAL REFERENCE MODEL VELOCITY/1(u_cmd)
  [v_des] -> INTERNAL REFERENCE MODEL VELOCITY/2(v_cmd)
  [w_des] -> INTERNAL REFERENCE MODEL VELOCITY/3(w_cmd)
  [Phi_cmd] -> Scope12/1, INTERNAL REFERENCE MODEL ATTITUDE/1(phi_cmd)
  [Theta_cmd] -> Scope12/2, Scope8/2, INTERNAL REFERENCE MODEL ATTITUDE/2(theta_cmd)  "command"
  [yaw_des] -> INTERNAL REFERENCE MODEL ATTITUDE/3(psi_cmd), Scope12/3
  Vector Concatenate/1 -> Scope1/1, [dv_inner]
  MATLAB Function/1(B_inner) -> Scope2/1, B_matrix/1, Pseudoinverse/1
  Pseudoinverse/1 -> MatrixMultiply/1, Scope4/1
  MatrixMultiply/1 -> Scope3/1, Sum8/1  "du"
  [omega_1] -> Vector Concatenate1/1
  [omega_2] -> Vector Concatenate1/2
  [omega_3] -> Vector Concatenate1/3
  [omega_4] -> Vector Concatenate1/4
  Vector Concatenate1/1 -> Sum7/2
  Constant2/1 -> Sum7/1
  Sum7/1 -> Sum8/2  "u"
  Sum8/1 -> Scope/1, Demux/1
  Demux/1 -> Motor_1_omega_input/1
  Demux/2 -> Motor_2_omega_input/1
  Demux/3 -> Motor_3_omega_input/1
  Demux/4 -> Motor_4_omega_input/1
  Sum4/1 -> Vector Concatenate/1
  Sum11/1 -> Vector Concatenate/2
  Sum13/1 -> Vector Concatenate/3
  [dv_inner] -> MatrixMultiply/2
  [T_increment] -> Gain/1
  Sum12/1 -> Sum19/1  "wd"
  Sum6/1 -> Sum18/1  "vd"
  Sum5/1 -> Sum17/1  "ud"
  Vector Concatenate3/1 -> Scope7/1, [dv_outer]
  [Vz_earth] -> vertical speed/1
  [Vy_earth] -> lateral speed/1
  [Vx_earth] -> horizontal speed/1
  Sum19/1 -> Vector Concatenate3/3
  Sum18/1 -> Vector Concatenate3/2
  Sum17/1 -> Vector Concatenate3/1
  [AxAyAz_earth] -> Demux3/1
  Demux3/3 -> Sum19/2
  Demux3/2 -> Sum18/2
  Demux3/1 -> Sum17/2
  [K_m] -> MATLAB Function/4(K_m)
  [Izz] -> MATLAB Function/3(Izz)
  [Iyy] -> MATLAB Function/2(Iyy)
  [Ixx] -> MATLAB Function/1(Ixx)
  [omega_3] -> MATLAB Function/8(Omega_3)
  [omega_1] -> MATLAB Function/6(Omega_1)
  [omega_4] -> MATLAB Function/9(Omega_4)
  [K_t] -> MATLAB Function/5(K_t)
  [b] -> MATLAB Function/10(b)
  [l] -> MATLAB Function/11(l)
  [omega_2] -> MATLAB Function/7(Omega_2)
  Pseudoinverse1/1 -> Scope11/1, MatrixMultiply1/1
  Sum20/1 -> [Phi_cmd]
  Demux5/1 -> Sum20/1
  [Phi] -> MATLAB Function1/2(Phi)
  Demux5/2 -> Sum16/1
  MatrixMultiply1/1 -> Demux5/1  "du"
  Sum21/1 -> Sum16/2  "u"
  [Theta] -> Sum21/2
  [m] -> MATLAB Function1/5(m)
  [T] -> MATLAB Function1/1(T)
  [dv_outer] -> MatrixMultiply1/2
  Constant1/1 -> Sum21/1
  [Phi] -> Sum15/2
  Sum16/1 -> [Theta_cmd]
  [Psi] -> MATLAB Function1/4(Psi)
  [Theta] -> MATLAB Function1/3(Theta)
  Demux5/3 -> [T_increment]
  Sum15/1 -> Sum20/2  "u"
  MATLAB Function1/1(B_outer) -> Pseudoinverse1/1, Display1/1, Scope9/1
  Constant3/1 -> Sum15/1
  INTERNAL REFERENCE MODEL ATTITUDE/4(pd_ref) -> ERROR CONTROLLER ATTITUDE/1(pd_ref)
  INTERNAL REFERENCE MODEL ATTITUDE/5(qd_ref) -> ERROR CONTROLLER ATTITUDE/2(qd_ref)
  INTERNAL REFERENCE MODEL ATTITUDE/6(rd_ref) -> ERROR CONTROLLER ATTITUDE/3(rd_ref)
  INTERNAL REFERENCE MODEL ATTITUDE/7(p_ref) -> ERROR CONTROLLER ATTITUDE/4(p_ref)
  INTERNAL REFERENCE MODEL ATTITUDE/8(q_ref) -> ERROR CONTROLLER ATTITUDE/5(q_ref)
  INTERNAL REFERENCE MODEL ATTITUDE/9(r_ref) -> ERROR CONTROLLER ATTITUDE/6(r_ref)
  INTERNAL REFERENCE MODEL ATTITUDE/10(phi_ref) -> ERROR CONTROLLER ATTITUDE/7(phi_ref)
  INTERNAL REFERENCE MODEL ATTITUDE/11(theta_ref) -> Scope8/1, ERROR CONTROLLER ATTITUDE/8(theta_ref)  "reference"
  INTERNAL REFERENCE MODEL ATTITUDE/12(psi_ref) -> ERROR CONTROLLER ATTITUDE/9(psi_ref)
  INTERNAL REFERENCE MODEL ATTITUDE/1(pdd_ref) -> Sum4/1
  INTERNAL REFERENCE MODEL ATTITUDE/2(qdd_ref) -> Sum11/1
  INTERNAL REFERENCE MODEL ATTITUDE/3(rdd_ref) -> Sum13/1
  ERROR CONTROLLER ATTITUDE/1(pdd_ec) -> Sum4/2
  ERROR CONTROLLER ATTITUDE/2(qdd_ec) -> Sum11/2
  ERROR CONTROLLER ATTITUDE/3(rdd_ec) -> Sum13/2
  Constant/1 -> MATLAB Function/12(K_act_inner)
  Gain/1 -> Vector Concatenate/4
  [Vz_earth] -> Scope5/2  "w"
  [Theta] -> Scope8/3  "state"

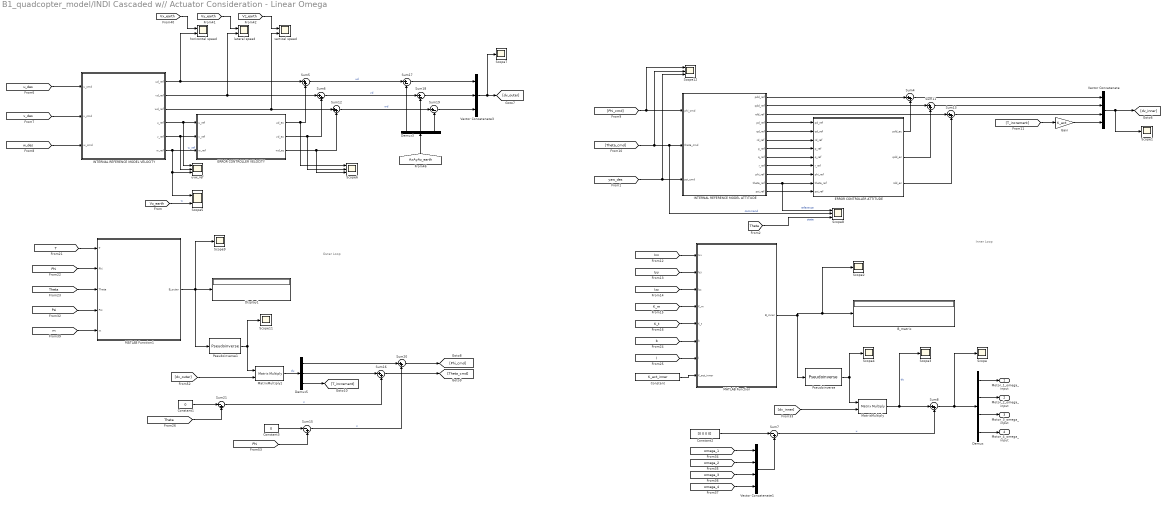
== system B1_quadcopter_model/INDI Cascaded w// Actuator Consideration - Linear Omega ==
  note: Outer Loop
  note: Inner Loop
  B_matrix : Display
  Constant : Constant  Value=K_act_inner
  Constant1 : Constant  Value=0
  Constant2 : Constant  Value=[0 0 0 0]
  Constant3 : Constant  Value=0
  Demux : Demux
  Demux3 : Demux  Outputs=3
  Demux5 : Demux  Outputs=3
  Display1 : Display
  ERROR CONTROLLER ATTITUDE : Subsystem
  ERROR CONTROLLER VELOCITY : Subsystem
  Gain : Gain  Gain=K_act
  INTERNAL REFERENCE MODEL ATTITUDE : Subsystem
  INTERNAL REFERENCE MODEL VELOCITY : Subsystem
  MATLAB Function : MATLAB Function  TreatAsAtomicUnit=on
  MATLAB Function1 : MATLAB Function  TreatAsAtomicUnit=on
  MatrixMultiply : Product  Multiplication=Matrix(*)
  MatrixMultiply1 : Product  Multiplication=Matrix(*)
  Pseudoinverse : dspinverses/Pseudoinverse  wanterr=off  SimulateUsing=Interpreted execution
      settings: SourceProductBaseCode=DS
  Pseudoinverse1 : dspinverses/Pseudoinverse  wanterr=off  SimulateUsing=Interpreted execution
      settings: SourceProductBaseCode=DS
  Scope{,1..4,7,9,11} (8 alike) : Scope
  Scope12 : Scope  NumInputPorts=3
  Scope5 : Scope  NumInputPorts=2
  Scope6 : Scope  NumInputPorts=3
  Scope8 : Scope  NumInputPorts=3
  Sum{4..6,8,11..13,16,20} (9 alike) : Sum  Inputs=|++
  Sum15 : Sum  Inputs=|-+
  Sum17 : Sum  Inputs=|+-
  Sum18 : Sum  Inputs=|+-
  Sum19 : Sum  Inputs=|+-
  Sum21 : Sum  Inputs=|-+
  Sum7 : Sum  Inputs=|-+
  Vector Concatenate : Concatenate  NumInputs=4
  Vector Concatenate1 : Concatenate  NumInputs=4
  Vector Concatenate3 : Concatenate  NumInputs=3
  horizontal speed : Scope  NumInputPorts=2
  lateral speed : Scope  NumInputPorts=2
  uvw_ref : Scope  NumInputPorts=3
  vertical speed : Scope  NumInputPorts=2
  Motor_1_omega_input : Outport
  Motor_2_omega_input : Outport  Port=2
  Motor_3_omega_input : Outport  Port=3
  Motor_4_omega_input : Outport  Port=4
  wires:
  ERROR CONTROLLER VELOCITY/1(ud_ec) -> Sum5/2, Scope6/1
  ERROR CONTROLLER VELOCITY/3(wd_ec) -> Sum12/2, Scope6/3
  INTERNAL REFERENCE MODEL VELOCITY/3(wd_ref) -> vertical speed/2, Sum12/1
  INTERNAL REFERENCE MODEL VELOCITY/2(vd_ref) -> lateral speed/2, Sum6/1
  INTERNAL REFERENCE MODEL VELOCITY/5(v_ref) -> ERROR CONTROLLER VELOCITY/2(v_ref), uvw_ref/2
  INTERNAL REFERENCE MODEL VELOCITY/6(w_ref) -> ERROR CONTROLLER VELOCITY/3(w_ref), Scope5/1, uvw_ref/3  "w_ref"
  INTERNAL REFERENCE MODEL VELOCITY/1(ud_ref) -> horizontal speed/2, Sum5/1
  ERROR CONTROLLER VELOCITY/2(vd_ec) -> Sum6/2, Scope6/2
  INTERNAL REFERENCE MODEL VELOCITY/4(u_ref) -> ERROR CONTROLLER VELOCITY/1(u_ref), uvw_ref/1
  [u_des] -> INTERNAL REFERENCE MODEL VELOCITY/1(u_cmd)
  [v_des] -> INTERNAL REFERENCE MODEL VELOCITY/2(v_cmd)
  [w_des] -> INTERNAL REFERENCE MODEL VELOCITY/3(w_cmd)
  [Phi_cmd] -> Scope12/1, INTERNAL REFERENCE MODEL ATTITUDE/1(phi_cmd)
  [Theta_cmd] -> Scope12/2, Scope8/2, INTERNAL REFERENCE MODEL ATTITUDE/2(theta_cmd)  "command"
  [yaw_des] -> INTERNAL REFERENCE MODEL ATTITUDE/3(psi_cmd), Scope12/3
  Vector Concatenate/1 -> Scope1/1, [dv_inner]
  MATLAB Function/1(B_inner) -> Scope2/1, B_matrix/1, Pseudoinverse/1
  Pseudoinverse/1 -> MatrixMultiply/1, Scope4/1
  MatrixMultiply/1 -> Scope3/1, Sum8/1  "du"
  [omega_1] -> Vector Concatenate1/1
  [omega_2] -> Vector Concatenate1/2
  [omega_3] -> Vector Concatenate1/3
  [omega_4] -> Vector Concatenate1/4
  Vector Concatenate1/1 -> Sum7/2
  Constant2/1 -> Sum7/1
  Sum7/1 -> Sum8/2  "u"
  Sum8/1 -> Scope/1, Demux/1
  Demux/1 -> Motor_1_omega_input/1
  Demux/2 -> Motor_2_omega_input/1
  Demux/3 -> Motor_3_omega_input/1
  Demux/4 -> Motor_4_omega_input/1
  Sum4/1 -> Vector Concatenate/1
  Sum11/1 -> Vector Concatenate/2
  Sum13/1 -> Vector Concatenate/3
  [dv_inner] -> MatrixMultiply/2
  [T_increment] -> Gain/1
  Sum12/1 -> Sum19/1  "wd"
  Sum6/1 -> Sum18/1  "vd"
  Sum5/1 -> Sum17/1  "ud"
  Vector Concatenate3/1 -> Scope7/1, [dv_outer]
  [Vz_earth] -> vertical speed/1
  [Vy_earth] -> lateral speed/1
  [Vx_earth] -> horizontal speed/1
  Sum19/1 -> Vector Concatenate3/3
  Sum18/1 -> Vector Concatenate3/2
  Sum17/1 -> Vector Concatenate3/1
  [AxAyAz_earth] -> Demux3/1
  Demux3/3 -> Sum19/2
  Demux3/2 -> Sum18/2
  Demux3/1 -> Sum17/2
  [K_m] -> MATLAB Function/4(K_m)
  [Izz] -> MATLAB Function/3(Izz)
  [Iyy] -> MATLAB Function/2(Iyy)
  [Ixx] -> MATLAB Function/1(Ixx)
  [K_t] -> MATLAB Function/5(K_t)
  [b] -> MATLAB Function/6(b)
  [l] -> MATLAB Function/7(l)
  Pseudoinverse1/1 -> Scope11/1, MatrixMultiply1/1
  Sum20/1 -> [Phi_cmd]
  Demux5/1 -> Sum20/1
  [Phi] -> MATLAB Function1/2(Phi)
  Demux5/2 -> Sum16/1
  MatrixMultiply1/1 -> Demux5/1  "du"
  Sum21/1 -> Sum16/2  "u"
  [Theta] -> Sum21/2
  [m] -> MATLAB Function1/5(m)
  [T] -> MATLAB Function1/1(T)
  [dv_outer] -> MatrixMultiply1/2
  Constant1/1 -> Sum21/1
  [Phi] -> Sum15/2
  Sum16/1 -> [Theta_cmd]
  [Psi] -> MATLAB Function1/4(Psi)
  [Theta] -> MATLAB Function1/3(Theta)
  Demux5/3 -> [T_increment]
  Sum15/1 -> Sum20/2  "u"
  MATLAB Function1/1(B_outer) -> Pseudoinverse1/1, Display1/1, Scope9/1
  Constant3/1 -> Sum15/1
  INTERNAL REFERENCE MODEL ATTITUDE/4(pd_ref) -> ERROR CONTROLLER ATTITUDE/1(pd_ref)
  INTERNAL REFERENCE MODEL ATTITUDE/5(qd_ref) -> ERROR CONTROLLER ATTITUDE/2(qd_ref)
  INTERNAL REFERENCE MODEL ATTITUDE/6(rd_ref) -> ERROR CONTROLLER ATTITUDE/3(rd_ref)
  INTERNAL REFERENCE MODEL ATTITUDE/7(p_ref) -> ERROR CONTROLLER ATTITUDE/4(p_ref)
  INTERNAL REFERENCE MODEL ATTITUDE/8(q_ref) -> ERROR CONTROLLER ATTITUDE/5(q_ref)
  INTERNAL REFERENCE MODEL ATTITUDE/9(r_ref) -> ERROR CONTROLLER ATTITUDE/6(r_ref)
  INTERNAL REFERENCE MODEL ATTITUDE/10(phi_ref) -> ERROR CONTROLLER ATTITUDE/7(phi_ref)
  INTERNAL REFERENCE MODEL ATTITUDE/11(theta_ref) -> Scope8/1, ERROR CONTROLLER ATTITUDE/8(theta_ref)  "reference"
  INTERNAL REFERENCE MODEL ATTITUDE/12(psi_ref) -> ERROR CONTROLLER ATTITUDE/9(psi_ref)
  INTERNAL REFERENCE MODEL ATTITUDE/1(pdd_ref) -> Sum4/1
  INTERNAL REFERENCE MODEL ATTITUDE/2(qdd_ref) -> Sum11/1
  INTERNAL REFERENCE MODEL ATTITUDE/3(rdd_ref) -> Sum13/1
  ERROR CONTROLLER ATTITUDE/1(pdd_ec) -> Sum4/2
  ERROR CONTROLLER ATTITUDE/2(qdd_ec) -> Sum11/2
  ERROR CONTROLLER ATTITUDE/3(rdd_ec) -> Sum13/2
  Constant/1 -> MATLAB Function/8(K_act_inner)
  Gain/1 -> Vector Concatenate/4
  [Vz_earth] -> Scope5/2  "w"
  [Theta] -> Scope8/3  "state"

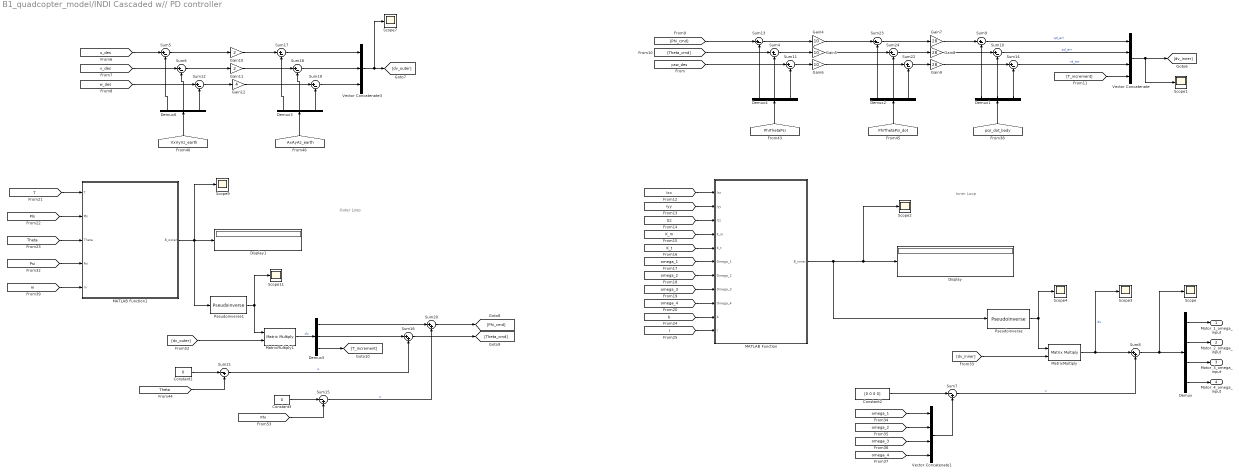
== system B1_quadcopter_model/INDI Cascaded w// PD controller ==
  note: Inner Loop
  note: Outer Loop
  Constant1 : Constant  Value=0
  Constant2 : Constant  Value=[0 0 0 0]
  Constant3 : Constant  Value=0
  Demux : Demux
  Demux{1..6} (6 alike) : Demux  Outputs=3
  Display : Display
  Display1 : Display
  Gain10 : Gain  Gain=2
  Gain11 : Gain  Gain=2
  Gain12 : Gain  Gain=4
  Gain4 : Gain  Gain=10
  Gain5 : Gain  Gain=10
  Gain6 : Gain  Gain=10
  Gain7 : Gain  Gain=28
  Gain8 : Gain  Gain=28
  Gain9 : Gain  Gain=28
  MATLAB Function : MATLAB Function  TreatAsAtomicUnit=on
  MATLAB Function1 : MATLAB Function  TreatAsAtomicUnit=on
  MatrixMultiply : Product  Multiplication=Matrix(*)
  MatrixMultiply1 : Product  Multiplication=Matrix(*)
  Pseudoinverse : dspinverses/Pseudoinverse  wanterr=off  SimulateUsing=Interpreted execution
      settings: SourceProductBaseCode=DS
  Pseudoinverse1 : dspinverses/Pseudoinverse  wanterr=off  SimulateUsing=Interpreted execution
      settings: SourceProductBaseCode=DS
  Scope{,1..4,7,9,11} (8 alike) : Scope
  Sum{4..6,9..14,17..19,22..24} (15 alike) : Sum  Inputs=|+-
  Sum15 : Sum  Inputs=|-+
  Sum16 : Sum  Inputs=|++
  Sum20 : Sum  Inputs=|++
  Sum21 : Sum  Inputs=|-+
  Sum7 : Sum  Inputs=|-+
  Sum8 : Sum  Inputs=|++
  Vector Concatenate : Concatenate  NumInputs=4
  Vector Concatenate1 : Concatenate  NumInputs=4
  Vector Concatenate3 : Concatenate  NumInputs=3
  Motor_1_omega_input : Outport
  Motor_2_omega_input : Outport  Port=2
  Motor_3_omega_input : Outport  Port=3
  Motor_4_omega_input : Outport  Port=4
  wires:
  Vector Concatenate/1 -> Scope1/1, [dv_inner]
  [Ixx] -> MATLAB Function/1(Ixx)
  [Iyy] -> MATLAB Function/2(Iyy)
  [Izz] -> MATLAB Function/3(Izz)
  [K_m] -> MATLAB Function/4(K_m)
  [K_t] -> MATLAB Function/5(K_t)
  [omega_1] -> MATLAB Function/6(Omega_1)
  [omega_2] -> MATLAB Function/7(Omega_2)
  [omega_3] -> MATLAB Function/8(Omega_3)
  [omega_4] -> MATLAB Function/9(Omega_4)
  [b] -> MATLAB Function/10(b)
  [l] -> MATLAB Function/11(l)
  MATLAB Function/1(B_inner) -> Pseudoinverse/1, Scope2/1, Display/1
  Pseudoinverse/1 -> MatrixMultiply/1, Scope4/1
  MatrixMultiply/1 -> Scope3/1, Sum8/1  "du"
  [omega_1] -> Vector Concatenate1/1
  [omega_2] -> Vector Concatenate1/2
  [omega_3] -> Vector Concatenate1/3
  [omega_4] -> Vector Concatenate1/4
  Vector Concatenate1/1 -> Sum7/2
  Constant2/1 -> Sum7/1
  Sum7/1 -> Sum8/2  "u"
  Sum8/1 -> Scope/1, Demux/1
  Demux/1 -> Motor_1_omega_input/1
  Demux/2 -> Motor_2_omega_input/1
  Demux/3 -> Motor_3_omega_input/1
  Demux/4 -> Motor_4_omega_input/1
  Sum9/1 -> Vector Concatenate/1  "qd_err"
  Sum10/1 -> Vector Concatenate/2  "pd_err"
  Sum14/1 -> Vector Concatenate/3  "rd_err"
  [pqr_dot_body] -> Demux1/1
  Demux1/3 -> Sum14/2
  Demux1/2 -> Sum10/2
  Demux1/1 -> Sum9/2
  [dv_inner] -> MatrixMultiply/2
  [T_increment] -> Vector Concatenate/4
  [dv_outer] -> MatrixMultiply1/2
  Constant3/1 -> Sum15/1
  MATLAB Function1/1(B_outer) -> Pseudoinverse1/1, Scope9/1, Display1/1
  Sum15/1 -> Sum20/2  "u"
  Pseudoinverse1/1 -> Scope11/1, MatrixMultiply1/1
  [T] -> MATLAB Function1/1(T)
  [Phi] -> MATLAB Function1/2(Phi)
  [Theta] -> MATLAB Function1/3(Theta)
  [Psi] -> MATLAB Function1/4(Psi)
  [m] -> MATLAB Function1/5(m)
  Vector Concatenate3/1 -> [dv_outer], Scope7/1
  Sum19/1 -> Vector Concatenate3/3
  Sum18/1 -> Vector Concatenate3/2
  Sum17/1 -> Vector Concatenate3/1
  [AxAyAz_earth] -> Demux3/1
  Demux3/3 -> Sum19/2
  Demux3/2 -> Sum18/2
  Demux3/1 -> Sum17/2
  [PhiThetaPsi] -> Demux4/1
  Demux4/2 -> Sum4/2
  Demux4/1 -> Sum13/2
  Demux4/3 -> Sum11/2
  [yaw_des] -> Sum11/1
  [Theta_cmd] -> Sum4/1
  [Phi_cmd] -> Sum13/1
  Sum11/1 -> Gain6/1
  Sum4/1 -> Gain5/1
  Sum13/1 -> Gain4/1
  MatrixMultiply1/1 -> Demux5/1  "du"
  Demux5/3 -> [T_increment]
  Demux5/2 -> Sum16/1
  Demux5/1 -> Sum20/1
  [Phi] -> Sum15/2
  Constant1/1 -> Sum21/1
  [Theta] -> Sum21/2
  Sum21/1 -> Sum16/2  "u"
  Sum20/1 -> [Phi_cmd]
  Sum16/1 -> [Theta_cmd]
  Gain4/1 -> Sum23/1
  Gain5/1 -> Sum24/1
  Demux2/3 -> Sum22/2
  Demux2/1 -> Sum23/2
  Gain6/1 -> Sum22/1
  Demux2/2 -> Sum24/2
  Sum23/1 -> Gain7/1
  Sum24/1 -> Gain8/1
  [PhiThetaPsi_dot] -> Demux2/1
  Sum22/1 -> Gain9/1
  Gain7/1 -> Sum9/1
  Gain8/1 -> Sum10/1
  Gain9/1 -> Sum14/1
  Demux6/1 -> Sum5/2
  Sum5/1 -> Gain10/1
  [VxVyVz_earth] -> Demux6/1
  Demux6/2 -> Sum6/2
  Demux6/3 -> Sum12/2
  Sum6/1 -> Gain11/1
  Sum12/1 -> Gain12/1
  Gain10/1 -> Sum17/1
  Gain11/1 -> Sum18/1
  Gain12/1 -> Sum19/1
  [u_des] -> Sum5/1
  [v_des] -> Sum6/1
  [w_des] -> Sum12/1
